simulink model "controlPosicion2PI"  (R2014a)
settings: Solver=ode45  StartTime=0.0  StopTime=10.0  RelTol=1e-3
libraries: simulink x1
settings Model: Creator=PedroBarquin  LastModifiedBy=PedroBarquin

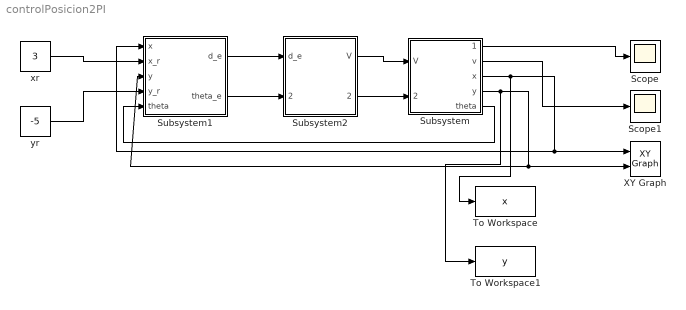
== system controlPosicion2PI ==
  Scope : Scope
  Scope1 : Scope
  Subsystem : Subsystem  mask{L=1, r=1, A=1, b=1, x_0=-2, y_0=3, omega_0=0}
  Subsystem1 : Subsystem
  Subsystem2 : Subsystem  mask{Kp_d=0.35, Kp_o=2, Kp_di=0.002, Kp_oi=0.5}
  To Workspace : ToWorkspace  VariableName=x  SaveFormat=Structure With Time  SampleTime=-1
  To Workspace1 : ToWorkspace  VariableName=y  SaveFormat=Structure With Time  SampleTime=-1
  XY Graph : simulink/Sinks/XY Graph  xmin=-7  xmax=7  ymin=-7  ymax=7  st=-1
  "xr " : Constant  Value=3
  "yr " : Constant  Value=-5
  wires:
  Subsystem/4("y ") -> To Workspace1/1, XY Graph/2, Subsystem1/3(y)
  Subsystem/3("x ") -> To Workspace/1, XY Graph/1, Subsystem1/1(x)
  Subsystem/2("v ") -> Scope1/1
  Subsystem/1("omega ") -> Scope/1
  Subsystem2/1(V) -> Subsystem/1("V ")
  Subsystem1/1(d_e) -> Subsystem2/1(d_e)
  Subsystem1/2("theta_e ") -> Subsystem2/2(theta_e)
  Subsystem2/2(" omega") -> Subsystem/2("omega ")
  Subsystem/5("theta ") -> Subsystem1/5("theta ")
  "xr "/1 -> Subsystem1/2("x_r ")
  "yr "/1 -> Subsystem1/4(y_r)

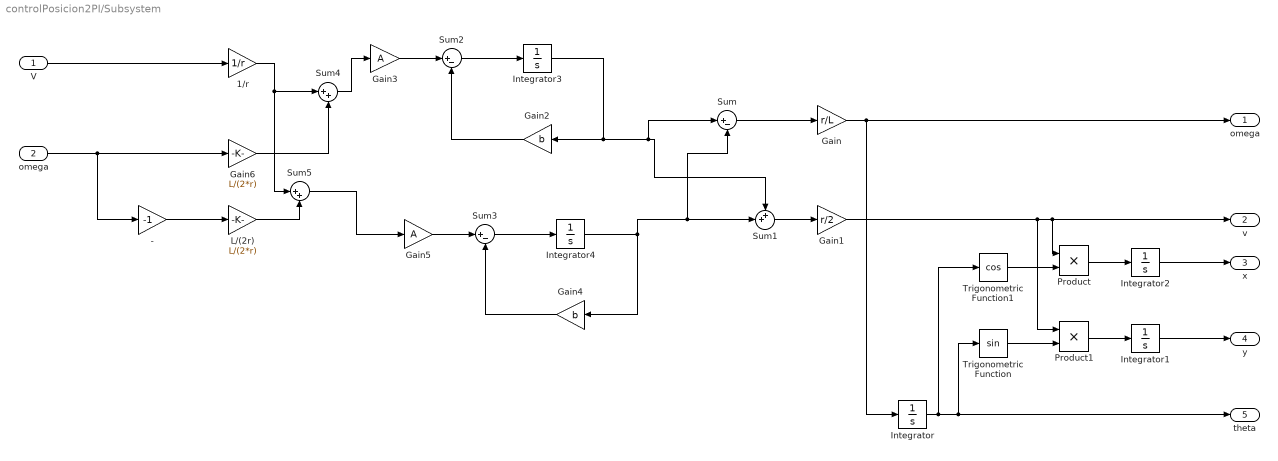
== system controlPosicion2PI/Subsystem ==
  "V " : Inport
  "omega " : Inport  Port=2
  "- " : Gain  Gain=-1
  1/r : Gain  Gain=1/r
  Gain : Gain  Gain=r/L
  Gain1 : Gain  Gain=r/2
  Gain2 : Gain  Gain=b
  Gain3 : Gain  Gain=A
  Gain4 : Gain  Gain=b
  Gain5 : Gain  Gain=A
  Gain6 : Gain  Gain=L/(2*r)
  Integrator : Integrator  InitialCondition=omega_0
  Integrator1 : Integrator  InitialCondition=y_0
  Integrator2 : Integrator  InitialCondition=x_0
  Integrator3 : Integrator  InitialCondition=omega_0
  Integrator4 : Integrator  InitialCondition=omega_0
  L/(2r) : Gain  Gain=L/(2*r)
  Product : Product
  Product1 : Product
  Sum : Sum  Inputs=|+-
  Sum1 : Sum  Inputs=++|
  Sum2 : Sum  Inputs=|+-
  Sum3 : Sum  Inputs=|+-
  Sum4 : Sum  Inputs=|++
  Sum5 : Sum  Inputs=|++
  Trigonometric Function : Trigonometry
  Trigonometric Function1 : Trigonometry  Operator=cos
  "omega " : Outport
  "v " : Outport  Port=2
  "x " : Outport  Port=3
  "y " : Outport  Port=4
  "theta " : Outport  Port=5
  wires:
  Sum2/1 -> Integrator3/1
  Gain3/1 -> Sum2/1
  Sum4/1 -> Gain3/1
  Gain2/1 -> Sum2/2
  Trigonometric Function/1 -> Product1/2
  Product/1 -> Integrator2/1
  Integrator2/1 -> "x "/1
  Gain/1 -> "omega "/1, Integrator/1
  Sum/1 -> Gain/1
  Integrator4/1 -> Gain4/1, Sum/2, Sum1/2
  Integrator3/1 -> Sum/1, Sum1/1, Gain2/1
  Sum1/1 -> Gain1/1
  Product1/1 -> Integrator1/1
  Gain1/1 -> Product1/1, "v "/1, Product/1
  Integrator/1 -> Trigonometric Function1/1, "theta "/1, Trigonometric Function/1
  Integrator1/1 -> "y "/1
  Trigonometric Function1/1 -> Product/2
  Gain5/1 -> Sum3/1
  Sum3/1 -> Integrator4/1
  Sum5/1 -> Gain5/1
  Gain4/1 -> Sum3/2
  "- "/1 -> L/(2r)/1
  1/r/1 -> Sum5/1, Sum4/1
  "omega "/1 -> "- "/1, Gain6/1
  Gain6/1 -> Sum4/2
  L/(2r)/1 -> Sum5/2
  "V "/1 -> 1/r/1

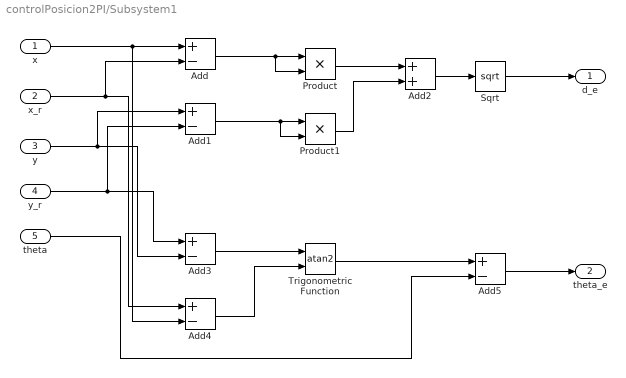
== system controlPosicion2PI/Subsystem1 ==
  x : Inport
  "x_r " : Inport  Port=2
  y : Inport  Port=3
  y_r : Inport  Port=4
  "theta " : Inport  Port=5
  Add{,1,3..5} (5 alike) : Sum  Inputs=+-
  Add2 : Sum
  Product : Product
  Product1 : Product
  Sqrt : Sqrt  SaturateOnIntegerOverflow=on
  Trigonometric Function : Trigonometry  Operator=atan2
  d_e : Outport
  "theta_e " : Outport  Port=2
  wires:
  Product1/1 -> Add2/2
  Add2/1 -> Sqrt/1
  Add5/1 -> "theta_e "/1
  Product/1 -> Add2/1
  Add3/1 -> Trigonometric Function/1
  Add1/1 -> Product1/2, Product1/1
  Add/1 -> Product/2, Product/1
  y/1 -> Add1/1, Add3/2
  y_r/1 -> Add1/2, Add3/1
  "x_r "/1 -> Add/2, Add4/1
  Sqrt/1 -> d_e/1
  x/1 -> Add/1, Add4/2
  Trigonometric Function/1 -> Add5/1
  Add4/1 -> Trigonometric Function/2
  "theta "/1 -> Add5/2

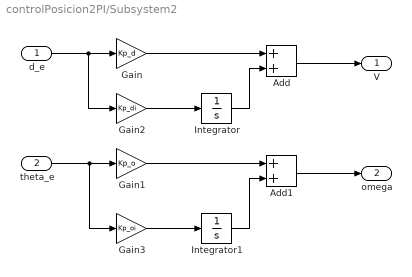
== system controlPosicion2PI/Subsystem2 ==
  d_e : Inport
  theta_e : Inport  Port=2
  Add : Sum
  Add1 : Sum
  Gain : Gain  Gain=Kp_d
  Gain1 : Gain  Gain=Kp_o
  Gain2 : Gain  Gain=Kp_di
  Gain3 : Gain  Gain=Kp_oi
  Integrator : Integrator
  Integrator1 : Integrator
  V : Outport
  " omega" : Outport  Port=2
  wires:
  theta_e/1 -> Gain3/1, Gain1/1
  d_e/1 -> Gain2/1, Gain/1
  Gain2/1 -> Integrator/1
  Gain3/1 -> Integrator1/1
  Integrator1/1 -> Add1/2
  Gain1/1 -> Add1/1
  Gain/1 -> Add/1
  Integrator/1 -> Add/2
  Add/1 -> V/1
  Add1/1 -> " omega"/1
